simulink model "H2_DRI_plant"  (R2023b)
settings: Solver=ode15s  StartTime=0.0  StopTime=3600*24*5
values from neighbouring files (symbols this model uses):
  a_b = 6*(1-eps_bed)/(r_p*2)    (= 200)    [H2_DRI_plant_loader.m]
  A_furnace = pi*r_furnace^2    (= 23.7582944428)    [H2_DRI_plant_loader.m]
  A_furnace_pel = A_furnace*(1-eps_bed)    (= 11.8791472214)    [H2_DRI_plant_loader.m]
  A_wall = (2*pi*r_furnace*dz)    (= 1.1674837564)    [H2_DRI_plant_loader.m]
  c_CH4init = interp1([1:1:length(c_CH4init)],c_CH4init, linspace(1,length(c_CH4init),n_furnace))    [H2_DRI_plant_loader.m]    (also in inital_conditions.m = out.CH4_conc.data(end,:); initcond_H2.mat = [9.94099064213e-45 -4.26076213273e-25 -4.27813906239e-25 -4.; initcond_H2_PEM.mat = [4.30667282687e-45 4.29087427587e-45 3.8700760922e-45 3.7994)
  c_Cinit = interp1([1:1:length(c_Cinit)],c_Cinit, linspace(1,length(c_Cinit),n_furnace))    [H2_DRI_plant_loader.m]    (also in inital_conditions.m = out.C_conc.data(end,:); initcond_H2.mat = [1.45956980986e-305 6.99081092012e-307 8.03725154841e-309 -3; initcond_H2_PEM.mat = [1.92191536232e-321 1.91203404941e-321 1.97132192691e-321 1.)
  c_CO2init = interp1([1:1:length(c_CO2init)],c_CO2init, linspace(1,length(c_CO2init),n_furnace))    [H2_DRI_plant_loader.m]    (also in inital_conditions.m = out.CO2_conc.data(end,:); initcond_H2.mat = [1.40671287015e-53 9.99429922421e-25 1.00349747704e-24 1.007; initcond_H2_PEM.mat = [4.30579616214e-45 4.28998535938e-45 3.86916279543e-45 3.798)
  c_COinit = interp1([1:1:length(c_COinit)],c_COinit, linspace(1,length(c_COinit),n_furnace))    [H2_DRI_plant_loader.m]    (also in inital_conditions.m = out.CO_conc.data(end,:); initcond_H2.mat = [8.62168160047e-54 2.62488347241e-25 2.63562031881e-25 2.646; initcond_H2_PEM.mat = [-1.41770643933e-43 -1.41248114323e-43 -1.27321677334e-43 -1)
  c_Fe2O3init = interp1([1:1:length(c_Fe2O3init)],c_Fe2O3init, linspace(1,length(c_Fe2O3init),n_furnace))    [H2_DRI_plant_loader.m]    (also in inital_conditions.m = out.Fe2O3_conc.data(end,:); initcond_H2.mat = [-0.0576294325141 -0.0562977053664 -0.0549879883395 -0.05369; initcond_H2_PEM.mat = [-0.0421766495112 -0.0410731169681 -0.0399918101679 -0.03893)
  c_Fe3O4init = interp1([1:1:length(c_Fe3O4init)],c_Fe3O4init, linspace(1,length(c_Fe3O4init),n_furnace))    [H2_DRI_plant_loader.m]    (also in inital_conditions.m = out.Fe3O4_conc.data(end,:); initcond_H2.mat = [0.0460784397936 0.0452182842983 0.0443654100081 0.043519007; initcond_H2_PEM.mat = [0.0345314201173 0.0338401633931 0.0331554273597 0.032476466)
  c_Feinit = interp1([1:1:length(c_Feinit)],c_Feinit, linspace(1,length(c_Feinit),n_furnace))    [H2_DRI_plant_loader.m]    (also in inital_conditions.m = out.Fe_conc.data(end,:); initcond_H2.mat = [2291.15615825 2257.57098555 2219.35021937 2176.85237423 213; initcond_H2_PEM.mat = [2291.15370188 2257.40533074 2219.07663621 2176.56351656 213)
  c_FeOinit = interp1([1:1:length(c_FeOinit)],c_FeOinit, linspace(1,length(c_FeOinit),n_furnace))    [H2_DRI_plant_loader.m]    (also in inital_conditions.m = out.FeO_conc.data(end,:); initcond_H2.mat = [120.587032003 163.793602795 212.96382844 267.636483226 327.; initcond_H2_PEM.mat = [120.587036941 164.003608886 213.312732219 268.005087273 327)
  c_H2init = interp1([1:1:length(c_H2init)],c_H2init, linspace(1,length(c_H2init),n_furnace))    [H2_DRI_plant_loader.m]    (also in inital_conditions.m = out.H2_conc.data(end,:); initcond_H2.mat = [22.889073739 22.8842667021 22.8746324515 22.8599710419 22.8; initcond_H2_PEM.mat = [17.1469199078 17.1645959742 17.1787956185 17.1891948084 17.)
  c_H2Oinit = interp1([1:1:length(c_H2Oinit)],c_H2Oinit, linspace(1,length(c_H2Oinit),n_furnace))    [H2_DRI_plant_loader.m]    (also in inital_conditions.m = out.H2O_conc.data(end,:); initcond_H2.mat = [2.19324064628 2.2939246227 2.40633645516 2.52967076126 2.66; initcond_H2_PEM.mat = [0.652099757837 0.728496202531 0.813916572535 0.907739128718)
  c_N2init = interp1([1:1:length(c_N2init)],c_N2init, linspace(1,length(c_N2init),n_furnace))    [H2_DRI_plant_loader.m]    (also in inital_conditions.m = out.N2_conc.data(end,:); initcond_H2.mat = [0.439764167248 0.441445162144 0.443247144888 0.445152489232; initcond_H2_PEM.mat = [0.271051060899 0.272483637209 0.274000693264 0.275587826454)
  CCeaf = CC_eaf*TPDls*365    (= 195258297.6)    [H2_DRI_plant_loader.m]
  CCelect = CC_elect*MWelect*1000    (= 420000000)    [H2_DRI_plant_loader.m]
  CCsf = 49080*(TPDls*DRIsteel_conv/24*1000)^(0.6538)    (= 108365944.556)    [H2_DRI_plant_loader.m]
  CO2_diff_prop = [MM_CO2, 26.9]    [H2_DRI_plant_loader.m]
  CO_diff_prop = [MM_CO, 18.9]    [H2_DRI_plant_loader.m]
  dz = (h_furnace/(n_furnace-1))    (= 0.0675675675676)    [H2_DRI_plant_loader.m]
  eps_bed = 0.5    [H2_DRI_plant_loader.m]
  H2_diff_prop = [MM_H2, 2.31*2]    [H2_DRI_plant_loader.m]
  H2O_diff_prop = [MM_H2O, 13.1]    [H2_DRI_plant_loader.m]
  H2only = true    [H2_DRI_plant_loader.m]
  I_metal = P_metal/tau_metal    (= -0.00212856534696)    [H2_DRI_plant_loader.m]
  I_temp = P_metal/tau_temp    (= -0.00681140911026)    [H2_DRI_plant_loader.m]
  Kd = 5.29e-4    (= 0.000529)    [H2_DRI_plant_loader.m]
  Kmetal = -0.0435    [H2_DRI_plant_loader.m]
  MM_C = 12.011/1000    (= 0.012011)    [H2_DRI_plant_loader.m]
  MM_CH4 = 16.04    [H2_DRI_plant_loader.m]
  MM_CO = 28.01    [H2_DRI_plant_loader.m]
  MM_CO2 = 44.01    [H2_DRI_plant_loader.m]
  MM_Fe = 55.845/1000    (= 0.055845)    [H2_DRI_plant_loader.m]    (also in iron_props.m)
  MM_Fe2O3 = 159.69/1000    (= 0.15969)    [H2_DRI_plant_loader.m]    (also in iron_props.m)
  MM_Fe3O4 = 231.53/1000    (= 0.23153)    [H2_DRI_plant_loader.m]    (also in iron_props.m = 0.25153)
  MM_FeO = 71.844/1000    (= 0.071844)    [H2_DRI_plant_loader.m]    (also in iron_props.m)
  MM_H2 = 2.016    [H2_DRI_plant_loader.m]
  MM_H2O = 18.015    [H2_DRI_plant_loader.m]
  MM_N2 = 28.013    [H2_DRI_plant_loader.m]
  n_furnace = 75    [H2_DRI_plant_loader.m]
  ndotin = 2078.874    [H2_DRI_plant_loader.m]
  nr1init = interp1([1:1:length(nr1init)],nr1init, linspace(1,length(nr1init),n_furnace))    [H2_DRI_plant_loader.m]    (also in inital_conditions.m = out.nr1.data(end,:); initcond_H2.mat = [17138.9259823 17138.9192887 17138.9127057 17138.9062259 171; initcond_H2_PEM.mat = [17138.8483125 17138.8427658 17138.8373309 17138.8319998 171)
  nr2init = interp1([1:1:length(nr2init)],nr2init, linspace(1,length(nr2init),n_furnace))    [H2_DRI_plant_loader.m]    (also in inital_conditions.m = out.nr2.data(end,:); initcond_H2.mat = [11425.7909148 11425.7894343 11425.7880023 11425.7866166 114; initcond_H2_PEM.mat = [11425.7791649 11425.7778635 11425.776614 11425.7754137 1142)
  nr3init = interp1([1:1:length(nr3init)],nr3init, linspace(1,length(nr3init),n_furnace))    [H2_DRI_plant_loader.m]    (also in inital_conditions.m = out.nr3.data(end,:); initcond_H2.mat = [32930.1678524 32447.4572478 31898.1205118 31287.3104766 306; initcond_H2_PEM.mat = [32930.1325476 32445.0763361 31894.188375 31283.1588034 3061)
  P_gin = 101325*1.8    (= 182385)    [H2_DRI_plant_loader.m]
  P_metal = tau_metal/(Kmetal*tau_metal_desired)    (= -24.5210727969)    [H2_DRI_plant_loader.m]
  P_temp = tau_temp/(Kmetal*tau_temp_desired)    (= -45.9770114943)    [H2_DRI_plant_loader.m]
  R = 8.314    [Bou.m]    (also in H2_DRI_plant_loader.m; MD.m; SMR.m; USCM_CO.m)
  r_furnace = 2.75    [H2_DRI_plant_loader.m]
  r_p = 15e-3/2    (= 0.0075)    [H2_DRI_plant_loader.m]
  rho_p = 3528    [H2_DRI_plant_loader.m]
  Solids_In_Flow = 44.1    [H2_DRI_plant_loader.m]
  T_gin = 947 + 273    (= 1220)    [H2_DRI_plant_loader.m]
  T_ginit = interp1([1:1:length(T_ginit)],T_ginit, linspace(1,length(T_ginit),n_furnace))    [H2_DRI_plant_loader.m]    (also in inital_conditions.m = out.T_g.data(end,2:end); initcond_H2.mat = [1193.47241077 1188.60147936 1183.4413554 1178.04610025 1172; initcond_H2_PEM.mat = [1213.62674902 1206.86882145 1199.80656651 1192.51337179 118)
  T_sin = -10 + 273    (= 263)    [H2_DRI_plant_loader.m]
  T_sinit = interp1([1:1:length(T_sinit)],T_sinit, linspace(1,length(T_sinit),n_furnace))    [H2_DRI_plant_loader.m]    (also in inital_conditions.m = out.T_s.data(end,1:end-1); initcond_H2.mat = [1188.32225462 1183.11411515 1177.66723955 1172.0331792 1166; initcond_H2_PEM.mat = [1207.76768382 1200.67884676 1193.34151616 1185.82650883 117)
  tau = 1    [H2_DRI_plant_loader.m]
  tau_d = 3600*2    (= 7200)    [H2_DRI_plant_loader.m]
  tau_metal = 3.2*3600    (= 11520)    [H2_DRI_plant_loader.m]
  V_g = (4/3)*pi*r_p^3*n_pellets_dz*(eps_bed/(1-eps_bed))    (= 0.802645082526)    [H2_DRI_plant_loader.m]
  V_p = 4/3*pi*r_p^3    (= 1.76714586764e-06)    [H2_DRI_plant_loader.m]
  V_s = (4/3)*pi*r_p^3*n_pellets_dz    (= 0.802645082526)    [H2_DRI_plant_loader.m]
  w_Cin = 0    [H2_DRI_plant_loader.m]
  w_Fe2O3in = 0.9665    [H2_DRI_plant_loader.m]
  w_Fe3O4in = 0    [H2_DRI_plant_loader.m]
  w_Fein = 0    [H2_DRI_plant_loader.m]
  w_FeOin = 0    [H2_DRI_plant_loader.m]
  w_Ganin = 0.0335    [H2_DRI_plant_loader.m]
  x_CH4in = 0.105824828    [H2_DRI_plant_loader.m]
  x_CO2in = 0.024    [H2_DRI_plant_loader.m]
  x_COin = 0.320711862    [H2_DRI_plant_loader.m]
  x_H2in = 0.489526511    [H2_DRI_plant_loader.m]
  x_H2Oin = 0.042557156    [H2_DRI_plant_loader.m]
  x_N2in = 0.017379642    [H2_DRI_plant_loader.m]
libraries: slpidlib x3, simulink x1
(part 3 of 3)

== matlab function H2_DRI_plant/Wet Scrubber/MATLAB Function ==
  data: P_gin input; P_gout output; T_gout output; T_gin input; ndotin input; x_H2in input; x_H2Oin input; x_N2in input; x_COin input; x_CO2in input; x_CH4in input; ndotout output; x_H2out output; x_H2Oout output; x_N2out output; x_COout output; x_CO2out output; x_CH4out output; T_amb input
function [P_gout, T_gout, ndotout, x_H2out, x_H2Oout, x_N2out, x_COout, x_CO2out, x_CH4out] ...
    = scrubber(P_gin, T_gin, ndotin, x_H2in, x_H2Oin, x_N2in, x_COin, x_CO2in, x_CH4in, T_amb)

P_gout = P_gin - 0.25*101325; %Pa, estimate that lose 0.25 atm through scrubber

% 15 C/K above 
T_sat = T_amb + 15; % K, temp cooled down to 

% NIST WebBook - Stull 1947
% T in K
A = 4.6543;
B = 1435.264;
C = -64.848;

P_sat = 10^(A - B/(C+T_sat))*1e5; % bar converted to Pa

x_H2Oout = P_sat/P_gout;

ndotout = ndotin*(x_H2Oin-1)/(x_H2Oout-1);
ndot_H2O_removed = ndotin - ndotout;

T_gout = T_sat;

moles_H2 = ndotin*x_H2in;
moles_N2 = ndotin*x_N2in;
moles_CO = ndotin*x_COin;
moles_CO2 = ndotin*x_CO2in;
moles_CH4 = ndotin*x_CH4in;

x_H2out = moles_H2/ndotout;
x_N2out = moles_N2/ndotout;
x_COout = moles_CO/ndotout;
x_CO2out = moles_CO2/ndotout;
x_CH4out = moles_CH4/ndotout;

== matlab function H2_DRI_plant/Splitter/splitter ==
  data: ndotin input; purgefraction input; ndot_comp output; ndot_purge output
function [ndot_comp, ndot_purge] = splitter(ndotin, purgefraction)

ndot_purge = purgefraction*ndotin;
ndot_comp = ndotin*(1-purgefraction);

== matlab function H2_DRI_plant/Recycle Compressor/compressor ==
  data: P_g_sp input; P_gin input; P_gout output; T_gin input; T_gout output
function [P_gout, T_gout] = compressor(P_g_sp, P_gin, T_gin)

npoly = 1.4;

P_gout = P_g_sp;

T_gout = T_gin*(P_gout/P_gin)^((npoly-1)/npoly);

== matlab function H2_DRI_plant/Mixer/MATLAB Function ==
  data: P_gin_e input; P_gout output; T_gout output; T_gin_e input; ndotin_e input; x_H2in_e input; x_H2Oin_e input; x_N2in_e input; x_COin_e input; x_CO2in_e input; x_CH4in_e input; ndotout output; x_H2out output; x_H2Oout output; x_N2out output; x_COout output; x_CO2out output; x_CH4out output; P_gin_r input; T_gin_r input; ndotin_r input; x_H2in_r input; x_H2Oin_r input; x_N2in_r input; x_COin_r input; x_CO2in_r input; x_CH4in_r input
function [P_gout, T_gout, ndotout, x_H2out, x_H2Oout, x_N2out, x_COout, x_CO2out, x_CH4out] ...
    = scrubber(P_gin_e, T_gin_e, ndotin_e, x_H2in_e, x_H2Oin_e, x_N2in_e, x_COin_e, x_CO2in_e, x_CH4in_e,...
               P_gin_r, T_gin_r, ndotin_r, x_H2in_r, x_H2Oin_r, x_N2in_r, x_COin_r, x_CO2in_r, x_CH4in_r)

ndotout = ndotin_e + ndotin_r;

T_gout = T_gin_r; %need to update using specific heats

P_gout = (ndotin_e*P_gin_e + ndotin_r*P_gin_r)/(ndotout);

moles_H2 = ndotin_r*x_H2in_r + ndotin_e*x_H2in_e;
moles_H2O = ndotin_r*x_H2Oin_r + ndotin_e*x_H2Oin_e;
moles_N2 = ndotin_r*x_N2in_r + ndotin_e*x_N2in_e;
moles_CO = ndotin_r*x_COin_r+ ndotin_e*x_COin_e;
moles_CO2 = ndotin_r*x_CO2in_r + ndotin_e*x_CO2in_e;
moles_CH4 = ndotin_r*x_CH4in_r + ndotin_e*x_CH4in_e;

x_H2out = moles_H2/ndotout;
x_H2Oout = moles_H2O/ndotout;
x_N2out = moles_N2/ndotout;
x_COout = moles_CO/ndotout;
x_CO2out = moles_CO2/ndotout;
x_CH4out = moles_CH4/ndotout;

== matlab function H2_DRI_plant/DRI Shaft Furnace/Mixer/MATLAB Function ==
  data: P_gin_f input; P_gout output; T_gout output; T_gin_f input; ndotin_f input; x_H2in_f input; x_H2Oin_f input; x_N2in_f input; x_COin_f input; x_CO2in_f input; x_CH4in_f input; ndotout output; x_H2out output; x_H2Oout output; x_N2out output; x_COout output; x_CO2out output; x_CH4out output; ndotin_N2extra input
function [P_gout, T_gout, ndotout, x_H2out, x_H2Oout, x_N2out, x_COout, x_CO2out, x_CH4out] ...
    = mixer(P_gin_f, T_gin_f, ndotin_f, x_H2in_f, x_H2Oin_f, x_N2in_f, x_COin_f, x_CO2in_f, x_CH4in_f, ndotin_N2extra)

ndotout = ndotin_f + ndotin_N2extra;

T_gout = T_gin_f; %need to update using specific heats

P_gout = P_gin_f;

moles_H2 = ndotin_f*x_H2in_f;
moles_H2O = ndotin_f*x_H2Oin_f;
moles_N2 = ndotin_f*x_N2in_f + ndotin_N2extra;
moles_CO = ndotin_f*x_COin_f;
moles_CO2 = ndotin_f*x_CO2in_f;
moles_CH4 = ndotin_f*x_CH4in_f;

x_H2out = moles_H2/ndotout;
x_H2Oout = moles_H2O/ndotout;
x_N2out = moles_N2/ndotout;
x_COout = moles_CO/ndotout;
x_CO2out = moles_CO2/ndotout;
x_CH4out = moles_CH4/ndotout;

== matlab function H2_DRI_plant/Combustion Furnace/MATLAB Function ==
  data: ndot input; x_H2 input; x_H2O input; x_N2 input; x_CO input; x_CO2 input; x_CH4 input; T_g input; Q_heat output; T_gsp input; MM_H2O parameter; MM_H2 parameter; MM_N2 parameter; MM_CO parameter; MM_CO2 parameter; MM_CH4 parameter; mdot output; Cp_g output
function [Q_heat, mdot, Cp_g] = fcn(ndot, x_H2, x_H2O, x_N2, x_CO, x_CO2, x_CH4, T_g, T_gsp, MM_H2O, MM_H2, MM_N2, MM_CO, MM_CO2, MM_CH4)

T_g_mid = (T_g + T_gsp)/2;

mdot = ndot*(x_H2*MM_H2 + x_CO*MM_CO + x_H2O*MM_H2O +x_CO2*MM_CO2 + x_N2*MM_N2 + x_CH4*MM_CH4)/1000; %kg/s

% Weight fractions of each gas species
w_totin = (x_H2*MM_H2 + x_H2O*MM_H2O + x_N2*MM_N2 + x_CO*MM_CO + x_CO2*MM_CO2 +  x_CH4*MM_CH4);

w_H2in = x_H2*MM_H2/w_totin;
w_H2Oin = x_H2O*MM_H2O /w_totin;
w_N2in = x_N2*MM_N2/w_totin;
w_COin = x_CO*MM_CO/w_totin;
w_CO2in = x_CO2*MM_CO2/w_totin;
w_CH4in = x_CH4*MM_CH4/w_totin;

w_fracs = [w_H2in, w_H2Oin, w_N2in, w_COin, w_CO2in, w_CH4in]; % Create a vector of weight fractions for the prop_mix function

% Get properties from CoolProp interpolation based on temp of gas in
[rho_H2, mu_H2, k_H2, C_H2] = hydrogen(T_g_mid);
[rho_H2O, mu_H2O, k_H2O, C_H2O] = water(T_g_mid);
[rho_N2, mu_N2, k_N2, C_N2] = nitrogen(T_g_mid);
[rho_CO, mu_CO, k_CO, C_CO] = carbonmonoxide(T_g_mid);
[rho_CO2, mu_CO2, k_CO2, C_CO2] = carbondioxide(T_g_mid);
[rho_CH4, mu_CH4, k_CH4, C_CH4] = methane(T_g_mid);

% Create vectors of properties for prop_mix function
rhos = [rho_H2, rho_H2O, rho_N2, rho_CO, rho_CO2, rho_CH4];
mus = [mu_H2, mu_H2O, mu_N2, mu_CO, mu_CO2, mu_CH4];
ks = [k_H2, k_H2O, k_N2, k_CO, k_CO2, k_CH4];
Cps = [C_H2, C_H2O, C_N2, C_CO, C_CO2, C_CH4];

% get vicosicty and specific heat of gas mixture in
[~, ~, ~,  Cp_g] = prop_mix(rhos, mus, ks, Cps, w_fracs);

Q_heat = mdot*Cp_g*(T_gsp - T_g)/1e6;

== matlab function H2_DRI_plant/Combustion Furnace/MATLAB Function1 ==
  data: ndot_p input; Q_purge output; x_H2_p input
function Q_purge = purge_comb(ndot_p, x_H2_p)

Q_purge =  ndot_p*x_H2_p*238440/1e6;

== matlab function H2_DRI_plant/MATLAB Function ==
  data: MWelect input; LCOS output; MWng input; LCOE input; m_IO input; m_DRI input; CCeaf parameter; CCelect parameter; CCsf parameter; LCOS_io output; LCOS_elec output; LCOS_CC output
function [LCOS, LCOS_io, LCOS_elec, LCOS_CC] = LCOS(MWelect, MWng, LCOE, m_IO, m_DRI, CCeaf, CCelect, CCsf)


DRIsteel_conv = 1.075; %ratio of tonnes DRI to steel produced


m_steel = m_DRI/DRIsteel_conv/1000; %tonne/s steel


%==========================Capital Costs==============================

plant_lt = 20*8760*3600; %seconds, plant lifetime

%io_steelconv = 1.504 %ratio of tonnes of iron ore to steel produced


%==========================Labor==============================




%==========================Variable O&M==============================

cIO = 130/1000; % $/kg

io_cost = m_IO*cIO; % $/s, cost of iron ore
elec_cost = (MWelect)*LCOE/3600; % $/s, cost of electricity
%gas_cost = MWng*3.412*8760*CF*cNG; % $/yr, cost of ng




%% LCOS

CCtotal = CCeaf + CCelect + CCsf;
CCrate = CCtotal/plant_lt; % $/s for plant capital costs


LCOS = (io_cost + elec_cost + CCrate)/m_steel;

LCOS_io = (io_cost)/m_steel;
LCOS_elec = (elec_cost)/m_steel;
LCOS_CC = (CCrate)/m_steel;

%%

%lime and carbon costs
% carbon_consume = 27*ls_prod # kg, (kg/tonne ls * tonne_ls)
% lime_consume = 50*ls_prod # kg, (kg/tonne ls * tonne_ls)
% 
% carbon_cost = carbon_consume*180/1000 #$, cost of carbon
% lime_cost = lime_consume*100/1000
% 
% consumables = carbon_cost + lime_cost #cost of carbon and lime consumption
% 
% #stack replacement
% stack_cost = MWelect*8760*CF*0.975*stack_replace #0.975 is rectifier efficiency - cost to replace stacks

    
% #==========================Taxes and Insurance==============================
% CCannual = (CCsf + CCelect + CCeaf + BOP)*CRF
% 
% tx_insure = (CCannual)*0.02 #$/yr annual taxes and insurance
% tx_insure_h2 = (CCelect)*CRF*0.02
% 
% fix_LCOH2 = labor_elect + GA_elect + tx_insure_h2 #fixed op. cost for LCOH2
% 

% #==========================CO2 Emissions==============================
% 
% ng_CO2rate = 198 #kg CO2/MWh nat gas -from my 1st paper
% ng_CO2rate_us = 47 #kg CO2e nat upstream - from Incentives for Clean Hydrogen Production in the Inflation Reduction Act
% 
% lime_CO2rate = 0.05 #kg CO2/kg lime consumed
% carbon_CO2rate = 0.98 #kg CO2/kg carbon consumed
% io_CO2rate = 0.02 #kg CO2/kg iron ore
% pell_CO2rate = 0.16 #kg CO2/kg iron ore
% og_CO2rate = 0.101 #kg CO2/kg ls
% 
% elec_CO2 = (MWelect+MWeaf+MWboil+MWcomp)*8760*CF*elec_CO2rate #kg CO2/yr from electricity
% ng_CO2 = MWng*8760*CF*ng_CO2rate #kg CO2/yr from natural gas combustion
% 
% EAFog_CO2 = og_CO2rate*ls_prod*1000 #kg CO2/yr from combustion of EAF off gas
% 
% ng_CO2us = MWng*8760*CF*ng_CO2rate_us #kg CO2/yr from upstream natural gas use
% 
% lime_CO2 = lime_CO2rate*lime_consume #kg CO2/yr from lime production
% carbon_CO2 = carbon_CO2rate*carbon_consume #kg CO2/yr from coal/coke production
% io_CO2 = io_CO2rate*io_steelconv*TPDls*CF*365*1000 #kg CO2/yr from iron ore mining
% pell_CO2 = pell_CO2rate*io_steelconv*TPDls*CF*365*1000 #kg CO2/yr from iron ore pelletizing
% 
% mineralCO2 = lime_CO2 + carbon_CO2 + io_CO2 #kg CO2/yr from mineral production/mining excluding pelletizing
